simulink model "Independent"  (R2024a)
settings: Solver=VariableStepAuto  StartTime=0.0  StopTime=10.0  RelTol=1e-3
settings Model: Creator=이현민  LastModifiedBy=이현민

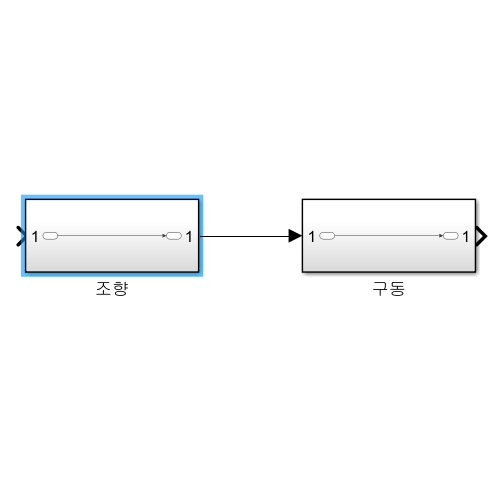
[thumbnail: Simulink's stored preview of the top-level diagram]
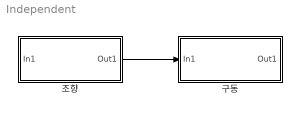
== system Independent ==
  구동 : Subsystem
  조향 : Subsystem
  wires:
  조향/1(Out1) -> 구동/1(In1)

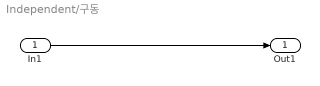
== system Independent/구동 ==
  In1 : Inport
  Out1 : Outport
  wires:
  In1/1 -> Out1/1

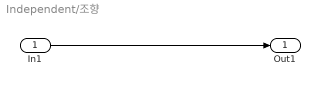
== system Independent/조향 ==
  In1 : Inport
  Out1 : Outport
  wires:
  In1/1 -> Out1/1
